simulink model "equalizer"  (R2023b)
settings: Solver=FixedStepAuto  StartTime=0.0  StopTime=10000  FixedStep=0.001  RelTol=1e-3
settings Model: Creator=Mahdi  LastModifiedBy=Mahdi
settings OptimizationCC: DefaultParameterBehavior=Inlined  OptimizeBlockIOStorage=off  BufferReuse=off  ReuseModelBlockBuffer=off  GlobalBufferReuse=off  ExpressionFolding=off  EnableMemcpy=off  PassReuseOutputArgsAs=Individual arguments  LocalBlockOutputs=off  ZeroExternalMemoryAtStartup=off  ZeroInternalMemoryAtStartup=off  OptimizeDataStoreBuffers=off  BusAssignmentInplaceUpdate=off  OptimizationLevel=level0  OptimizationCustomize=off  EfficientTunableParamExpr=on
settings DebuggingCC: ParameterTunabilityLossMsg=error
settings HardwareCC: ProdBitPerInt=16  ProdBitPerPointer=16  ProdBitPerSizeT=16  ProdBitPerPtrDiffT=16  ProdLargestAtomicFloat=None  ProdWordSize=16  ProdHWDeviceType=STMicroelectronics->ST10/Super10
settings SFSimCC: MATLABDynamicMemAlloc=off
settings RTWCC: Description=Embedded Coder  SystemTargetFile=ert.tlc  TemplateMakefile=ert_default_tmf  BuildConfiguration=Debug
settings CodeAppCC: ForceParamTrailComments=on  IgnoreCustomStorageClasses=off  OperatorAnnotations=on  SimulinkDataObjDesc=on  SFDataObjDesc=on  InsertBlockDesc=on
settings ERTTargetCC: TargetLangStandard=C99 (ISO)  GenerateSampleERTMain=on  SupportContinuousTime=on  SupportVariableSizeSignals=on  InlinedParameterPlacement=NonHierarchical  ERTCustomFileTemplate=example_file_process.tlc

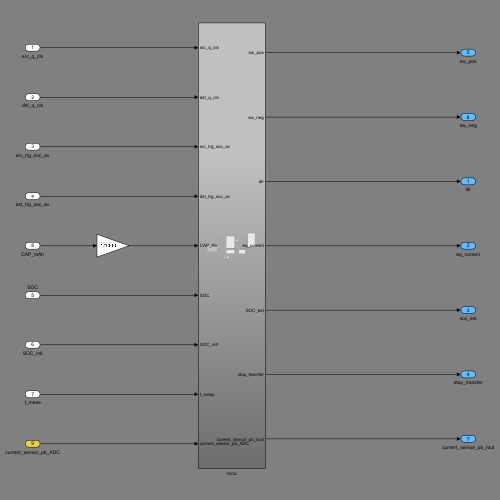
[thumbnail: Simulink's stored preview of the top-level diagram]
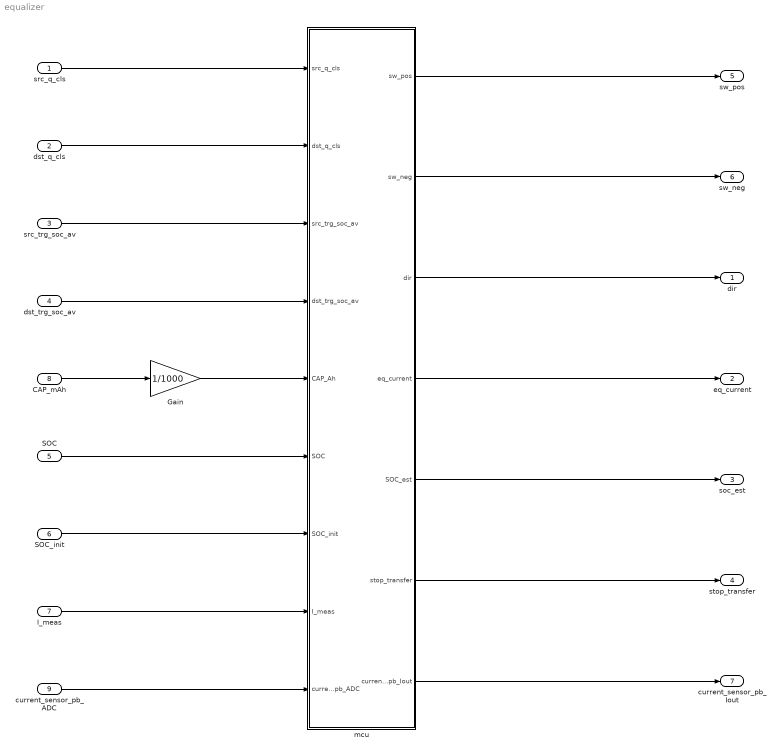
== system equalizer ==
  src_q_cls : Inport  PortDimensions=[1 2]
  dst_q_cls : Inport  Port=2  PortDimensions=[1 2]
  src_trg_soc_av : Inport  Port=3  PortDimensions=1
  dst_trg_soc_av : Inport  Port=4  PortDimensions=1
  SOC : Inport  Port=5  PortDimensions=[1 9]
  SOC_init : Inport  Port=6  PortDimensions=[1 9]
  I_meas : Inport  Port=7  PortDimensions=[1 9]
  CAP_mAh : Inport  Port=8  PortDimensions=[1 1]
  current_sensor_pb_ADC : Inport  Port=9  OutDataTypeStr=uint16
  Gain : Gain  Gain=1/1000
  mcu : Subsystem
  dir : Outport  OutDataTypeStr=int8
  eq_current : Outport  Port=2
  soc_est : Outport  Port=3  PortDimensions=[1 9]
  stop_transfer : Outport  Port=4  PortDimensions=1
  sw_pos : Outport  Port=5
  sw_neg : Outport  Port=6
  current_sensor_pb_Iout : Outport  Port=7
  wires:
  dst_q_cls/1 -> mcu/2(dst_q_cls)
  CAP_mAh/1 -> Gain/1
  dst_trg_soc_av/1 -> mcu/4(dst_trg_soc_av)
  src_trg_soc_av/1 -> mcu/3(src_trg_soc_av)
  src_q_cls/1 -> mcu/1(src_q_cls)
  I_meas/1 -> mcu/8(I_meas)
  mcu/4(eq_current) -> eq_current/1
  mcu/3(dir) -> dir/1
  mcu/5(SOC_est) -> soc_est/1
  Gain/1 -> mcu/5(CAP_Ah)
  mcu/6(stop_transfer) -> stop_transfer/1
  SOC_init/1 -> mcu/7(SOC_init)
  SOC/1 -> mcu/6(SOC)
  mcu/1(sw_pos) -> sw_pos/1
  mcu/2(sw_neg) -> sw_neg/1
  current_sensor_pb_ADC/1 -> mcu/9(current_sensor_pb_ADC)
  mcu/7(current_sensor_pb_Iout) -> current_sensor_pb_Iout/1

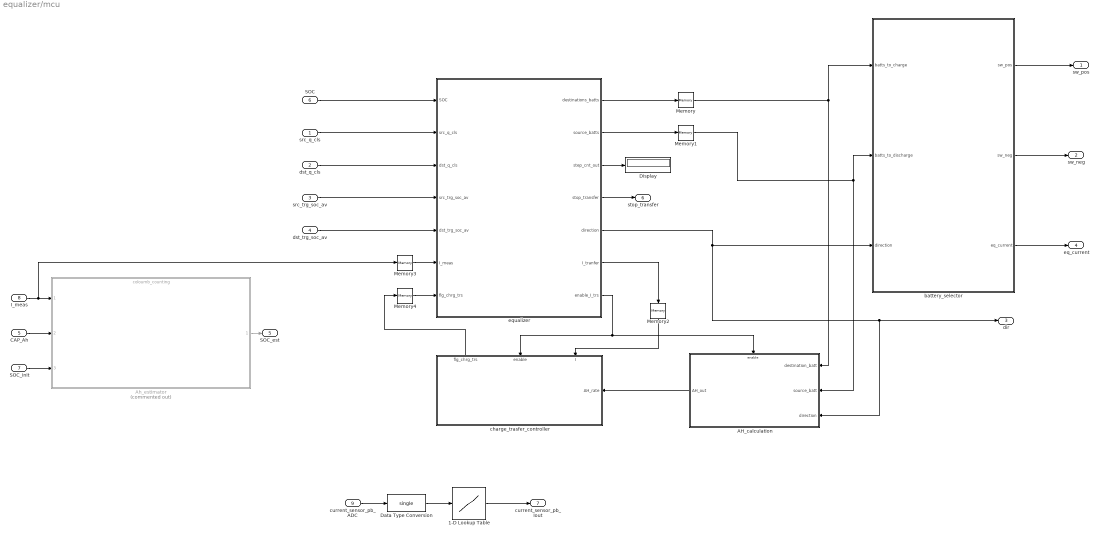
== system equalizer/mcu ==
  src_q_cls : Inport
  dst_q_cls : Inport  Port=2
  src_trg_soc_av : Inport  Port=3
  dst_trg_soc_av : Inport  Port=4
  CAP_Ah : Inport  Port=5
  SOC : Inport  Port=6
  SOC_init : Inport  Port=7
  I_meas : Inport  Port=8
  current_sensor_pb_ADC : Inport  Port=9
  1-D Lookup Table : Lookup_n-D  NumberOfTableDimensions=1  BreakpointsForDimension1=[52465 56650 58230]  BreakpointsForDimension1DataTypeStr=single  Table=[0 1042 1486]  TableDataTypeStr=single  IntermediateResultsDataTypeStr=single  InternalRulePriority=Speed  OutMin=0  OutMax=2000  OutDataTypeStr=single  RndMeth=Simplest  FractionDataTypeStr=single
  AH_calculation : Subsystem
  Ah_estimator : ModelReference  Commented=on  ModelNameDialog=coloumb_counting.slx  SimulationMode=Normal  ModelReferenceVersion=2.1
  Data Type Conversion : DataTypeConversion  OutDataTypeStr=single  SaturateOnIntegerOverflow=off  RndMeth=Floor
  Display : Display
  Memory{,1..4} (5 alike) : Memory
  battery_selector : MATLAB Function  TreatAsAtomicUnit=on
  charge_trasfer_controller : Subsystem
      settings: PortSchema="{\"entries\":[{\"content\":{\"sides\":[{\"content\":{},\"type\":\"ConnectorPlacement.EquallySpacedRectSide\",\"uuid\":\"48c70ec0-4261-4909-a719-c03e97c3e4ca\"},{\"content\":{\"connectorIds\":[\"In3\"],\"side\":\"RIGHT\"},\"type\":\"ConnectorPlacement.EquallySpacedRectSide\",\"uuid\":\"8a44a88a-c632-4005-90b8-1b0d09211c10\"},{\"content\":{\"connectorIds\":[\"Out1\",\"In1\",\"In2\"],\"side\":\"TOP\"},\"type\":\"ConnectorPlacement.EquallySpacedRectSide\",\"uuid\":\"71bafe47-820a-4a08-9919-e54bf550fba8\"}]},\"type\":\"ConnectorPlacement.EquallySpacedConnector\",\"uuid\":\"9c996bd2-099e-4131-a64b-67fbb4a72a45\"}],\"packageUris\":[\"http://schema.mathworks.com/mf0/Connector/R2020b\"],\"version\":\"1.0\"}"
  equalizer : MATLAB Function  TreatAsAtomicUnit=on
  sw_pos : Outport
  sw_neg : Outport  Port=2
  dir : Outport  Port=3
  eq_current : Outport  Port=4
  SOC_est : Outport  Port=5
  stop_transfer : Outport  Port=6
  current_sensor_pb_Iout : Outport  Port=7
  wires:
  Ah_estimator/1 -> SOC_est/1
  Memory3/1 -> equalizer/6(I_meas)
  AH_calculation/1(AH_out) -> charge_trasfer_controller/3(AH_rate)
  equalizer/2(source_batts) -> Memory1/1
  equalizer/4(stop_transfer) -> stop_transfer/1
  equalizer/7(enable_I_trs) -> AH_calculation/Enable, charge_trasfer_controller/1(enable)
  Memory2/1 -> charge_trasfer_controller/2(I)
  charge_trasfer_controller/1(flg_chrg_trs) -> Memory4/1
  Memory4/1 -> equalizer/7(flg_chrg_trs)
  src_q_cls/1 -> equalizer/2(src_q_cls)
  equalizer/5(direction) -> AH_calculation/3(direction), dir/1, battery_selector/3(direction)
  CAP_Ah/1 -> Ah_estimator/2
  equalizer/6(I_tranfer) -> Memory2/1
  SOC/1 -> equalizer/1(SOC)
  SOC_init/1 -> Ah_estimator/3
  battery_selector/2(sw_neg) -> sw_neg/1
  equalizer/1(destinations_batts) -> Memory/1
  I_meas/1 -> Memory3/1, Ah_estimator/1
  src_trg_soc_av/1 -> equalizer/4(src_trg_soc_av)
  dst_trg_soc_av/1 -> equalizer/5(dst_trg_soc_av)
  battery_selector/3(eq_current) -> eq_current/1
  battery_selector/1(sw_pos) -> sw_pos/1
  equalizer/3(step_cnt_out) -> Display/1
  Memory1/1 -> AH_calculation/2(source_batt), battery_selector/2(batts_to_discharge)
  Memory/1 -> AH_calculation/1(destination_batt), battery_selector/1(batts_to_charge)
  dst_q_cls/1 -> equalizer/3(dst_q_cls)
  current_sensor_pb_ADC/1 -> Data Type Conversion/1
  Data Type Conversion/1 -> 1-D Lookup Table/1
  1-D Lookup Table/1 -> current_sensor_pb_Iout/1

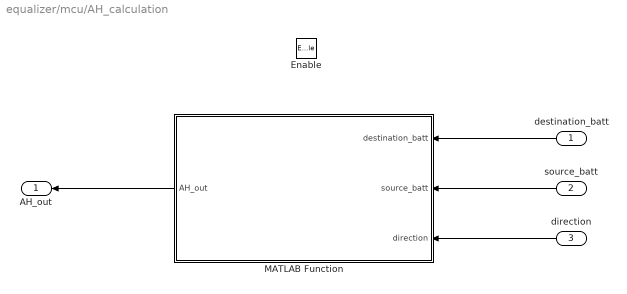
== system equalizer/mcu/AH_calculation ==
  destination_batt : Inport
  source_batt : Inport  Port=2
  direction : Inport  Port=3
  Enable : EnablePort
  MATLAB Function : MATLAB Function  TreatAsAtomicUnit=on
  AH_out : Outport
  wires:
  source_batt/1 -> MATLAB Function/2(source_batt)
  direction/1 -> MATLAB Function/3(direction)
  destination_batt/1 -> MATLAB Function/1(destination_batt)
  MATLAB Function/1(AH_out) -> AH_out/1

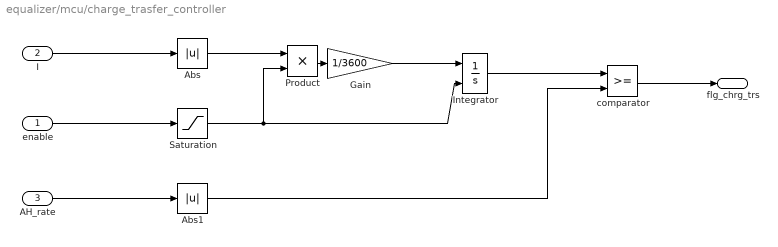
== system equalizer/mcu/charge_trasfer_controller ==
  enable : Inport
  I : Inport  Port=2
  AH_rate : Inport  Port=3
  Abs : Abs  SaturateOnIntegerOverflow=off
  Abs1 : Abs  SaturateOnIntegerOverflow=off
  Gain : Gain  Gain=1/3600
  Integrator : Integrator  ExternalReset=either
  Product : Product
  Saturation : Saturate  UpperLimit=1  LowerLimit=0
  comparator : RelationalOperator  OutDataTypeStr=boolean  RndMeth=Simplest  InputSameDT=off
  flg_chrg_trs : Outport
  wires:
  comparator/1 -> flg_chrg_trs/1
  AH_rate/1 -> Abs1/1
  Abs/1 -> Product/1
  Integrator/1 -> comparator/1
  Product/1 -> Gain/1
  enable/1 -> Saturation/1
  Gain/1 -> Integrator/1
  Saturation/1 -> Product/2, Integrator/2
  I/1 -> Abs/1
  Abs1/1 -> comparator/2

== matlab function equalizer/mcu/battery_selector ==
  data: batts_to_charge input; sw_pos output uint8; sw_neg output uint8; batts_to_discharge input; direction input; eq_current output
function [sw_pos, sw_neg, eq_current] = battery_selector(batts_to_charge, batts_to_discharge, direction)
    sw_pos = uint8(0);
    sw_neg = uint8(0);
    eq_current = 0;
    eq_current_tmp = 0;
% to prevent invalid switch selection
if ( batts_to_charge(1, 1) <= batts_to_charge(1, 2) && ...
     batts_to_discharge(1, 1) <= batts_to_discharge(1, 2))
    
    % charge the capacitor using batteries
    if(direction == 0)
        sw_pos = uint8(batts_to_discharge(1, 1));
        sw_neg = uint8(batts_to_discharge(1, 2));
        eq_current_tmp = 2;        
    % charge the battery using capacitor
    elseif(direction == 1)
        sw_pos = uint8(batts_to_charge(1, 1));
        sw_neg = uint8(batts_to_charge(1, 2));
        eq_current_tmp = 2;
    else
        sw_pos = uint8(0);
        sw_neg = uint8(0);
    end


    eq_current = eq_current_tmp;

end


end

== matlab function equalizer/mcu/equalizer ==
  settings: updateMethod=DISCRETE
  data: destinations_batts output; SOC input; source_batts output [..50]; src_q_cls input; dst_q_cls input; src_trg_soc_av input; dst_trg_soc_av input; I_meas input; step_cnt_out output; stop_transfer output; direction output int8; I_tranfer output; enable_I_trs output; flg_chrg_trs input
function [destinations_batts, source_batts, step_cnt_out, stop_transfer, direction, I_tranfer, enable_I_trs] = ...
    battery_selector ...
    (SOC, src_q_cls, dst_q_cls, src_trg_soc_av, dst_trg_soc_av, I_meas, flg_chrg_trs)


I_tranfer  = 0;
stop_transfer  = 0;
source_batts = [0 0];
destinations_batts = [0 0];
dst_trg_soc_av_tmp = dst_trg_soc_av;
src_trg_soc_av_tmp = src_trg_soc_av;

%dst_trg_soc_av_tmp(dst_trg_soc_av == 0) = Inf;
% src_trg_soc_av_tmp(src_trg_soc_av == 0) = Inf;
% the number of steps to equlalize the battery pack
step = length(src_q_cls);

persistent step_cnt;
persistent I_cells_source;
persistent I_cells_destination;
persistent dir;
persistent enable;



if isempty(step_cnt)
    step_cnt = 1;
    assert(1, 'Simulation terminated because x >= 10')

end

if isempty(I_cells_source)
    I_cells_source = 0;
end
if isempty(I_cells_destination)
    I_cells_destination = 0;
end
if isempty(dir)
    dir = int8(-1);
end
if isempty(enable)
    enable = 0;
end



soc = SOC';
if src_q_cls(1, :) > 0


    source_batts = src_q_cls(1, :);
    I_cells_source = I_meas(source_batts(1, 1));       % source cells current
    destinations_batts = dst_q_cls(1, :);
    I_cells_destination = I_meas(destinations_batts(1, 1));  % destication cells current



    if(dir == -1 && flg_chrg_trs == 0) % dischaege source if in the begining of charge transfering
        I_tranfer = I_cells_source;
        enable = 1; % start counting coulombs
        dir = int8(0); 
    end
    if(dir == 0)
        I_tranfer = I_cells_source;
    end

    if(dir == 0 && flg_chrg_trs == 1 && enable == 1) % reset the flag
        enable = 0;
    end

    if(dir == 0 && flg_chrg_trs == 0 && enable == 0) % charge the destination if the prevoius charge transfer terminated
        I_tranfer = I_cells_destination;
        enable = 1;
        dir = int8(1);
    end
    if(dir == 1)
        I_tranfer = I_cells_destination;
    end

    if(dir == 1 && flg_chrg_trs == 1 && enable == 1) % reset the flag
        enable = 0;
    end

    if(dir == 1 && flg_chrg_trs == 0 && enable == 0) % charge transfer terminated
        dir = int8(-1);
    end
    
    sm = mean(soc(src_q_cls(1, 1):src_q_cls(1, 2)));
    dm = mean(soc(dst_q_cls(1, 1):dst_q_cls(1, 2)));
    if(sm <= src_trg_soc_av_tmp(1) || dm >= dst_trg_soc_av_tmp(1)) && dir == -1
        stop_transfer = 1;
    end
else
    direction = int8(0);
    I_cells_source = 0;
    I_cells_destination = 0;
    dir = int8(-1);
    stop_transfer  = 1;
    enable = 0;
end
direction = int8(dir);
enable_I_trs = enable;


step_cnt_out = step_cnt;

end

== matlab function equalizer/mcu/AH_calculation/MATLAB Function ==
  data: destination_batt input; AH_out output; source_batt input; direction input
function AH_out = fcn(destination_batt, source_batt, direction)
AH_base = 0.001;
AH_coeff = 1;
AH_out = 0;

source_batt_number = source_batt(1, 2) - source_batt(1, 1) + 1;
destination_batt_number = destination_batt(1, 2) - destination_batt(1, 1) + 1;

if (source_batt_number > destination_batt_number)
    if direction == 0
        AH_coeff = destination_batt_number / source_batt_number;
    else
        AH_coeff = 1; 
    end
elseif source_batt_number < destination_batt_number
     if direction == 1
        AH_coeff = source_batt_number / destination_batt_number;
    else
        AH_coeff = 1; 
    end
end

AH_out = AH_base * AH_coeff;
